simulink model "sldemo_shared_data"  (R2019b)
settings: Solver=VariableStepAuto  StartTime=0.0  StopTime=14  RelTol=1e-3
undefined symbols (not defined in the file): I_gain, P_gain, setPt
settings Model: Creator=The MathWorks, Inc.  LastModifiedBy=bhisma
settings DataIOCC: SaveFormat=StructureWithTime  SaveState=on
settings DebuggingCC: ArithmeticOperatorsInVariantConditions=warning
settings SFSimCC: SimUseLocalCustomCode=off  CustomCodeUndefinedFunction=UseInterfaceOnly
settings RTWCC: RTWUseLocalCustomCode=off

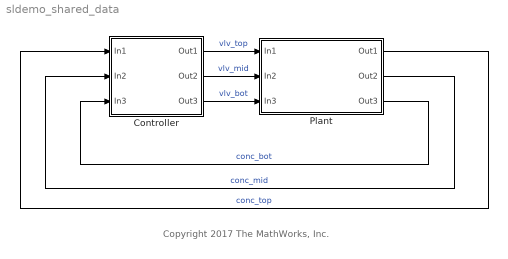
== system sldemo_shared_data ==
  note: Copyright 2017 The MathWorks, Inc.
  Controller : Subsystem
  Plant : Subsystem
  wires:
  Controller/1(Out1) -> Plant/1(In1)  "vlv_top"
  Controller/2(Out2) -> Plant/2(In2)  "vlv_mid"
  Controller/3(Out3) -> Plant/3(In3)  "vlv_bot"
  Plant/1(Out1) -> Controller/1(In1)  "conc_top"
  Plant/2(Out2) -> Controller/2(In2)  "conc_mid"
  Plant/3(Out3) -> Controller/3(In3)  "conc_bot"

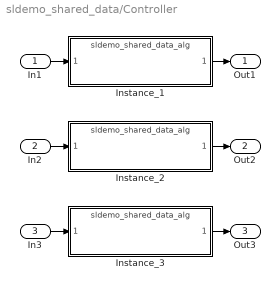
== system sldemo_shared_data/Controller ==
  In1 : Inport
  In2 : Inport  Port=2
  In3 : Inport  Port=3
  Instance_1 : ModelReference  ModelNameDialog=sldemo_shared_data_alg  ParameterArgumentNames=I_gain,P_gain,setPt  ParameterArgumentValues=1.31,0.98,1.8  UsingDefaultArgumentValue=0,0,0  SimulationMode=Normal  ModelReferenceVersion=1.121
  Instance_2 : ModelReference  ModelNameDialog=sldemo_shared_data_alg  ParameterArgumentNames=I_gain,P_gain,setPt  ParameterArgumentValues=1.18,0.98,2.3  UsingDefaultArgumentValue=0,0,0  SimulationMode=Normal  ModelReferenceVersion=1.121
  Instance_3 : ModelReference  ModelNameDialog=sldemo_shared_data_alg  ParameterArgumentNames=I_gain,P_gain,setPt  ParameterArgumentValues=0.98,1.12,1  UsingDefaultArgumentValue=0,0,0  SimulationMode=Normal  ModelReferenceVersion=1.121
  Out1 : Outport  VectorParamsAs1DForOutWhenUnconnected=off
  Out2 : Outport  Port=2  VectorParamsAs1DForOutWhenUnconnected=off
  Out3 : Outport  Port=3  VectorParamsAs1DForOutWhenUnconnected=off
  wires:
  Instance_1/1 -> Out1/1
  In3/1 -> Instance_3/1
  In1/1 -> Instance_1/1
  In2/1 -> Instance_2/1
  Instance_3/1 -> Out3/1
  Instance_2/1 -> Out2/1

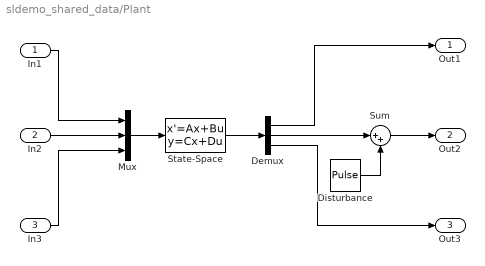
== system sldemo_shared_data/Plant ==
  In1 : Inport
  In2 : Inport  Port=2
  In3 : Inport  Port=3
  Demux : Demux  Outputs=3
  Disturbance : DiscretePulseGenerator  PulseType=Time based  Period=15  PhaseDelay=7.5
  Mux : Mux  Inputs=3
  State-Space : StateSpace  A=[-0.10002 0.00117 0.00173; -0.00981 -0.10002 0.00211; 0.00135 -0.00121 -0.09982]  B=[1.00130 -0.1423 0.0734; 0.1516 0.99945 -0.0946; -0.0734 0.1341 1.00002]  C=[0.99963 0.0115 0; 0 1.00001 0.0134; 0 0.0178 1.00050]  D=zeros(3,3)  InitialCondition=[1.80 2.3 1.00]
  Sum : Sum  Inputs=|++
  Out1 : Outport  VectorParamsAs1DForOutWhenUnconnected=off
  Out2 : Outport  Port=2  VectorParamsAs1DForOutWhenUnconnected=off
  Out3 : Outport  Port=3  VectorParamsAs1DForOutWhenUnconnected=off
  wires:
  In1/1 -> Mux/1
  In2/1 -> Mux/2
  In3/1 -> Mux/3
  Mux/1 -> State-Space/1
  State-Space/1 -> Demux/1
  Demux/1 -> Out1/1
  Demux/2 -> Sum/1
  Demux/3 -> Out3/1
  Sum/1 -> Out2/1
  Disturbance/1 -> Sum/2
